simulink library "pd_processing_lib"  (R2018b)
settings: Solver=VariableStepAuto  StartTime=0.0  StopTime=10.0  RelTol=1e-3
settings Model: Creator=Taylor  LastModifiedBy=Taylor

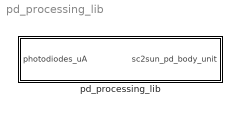
== system pd_processing_lib ==
  pd_processing_lib : Subsystem

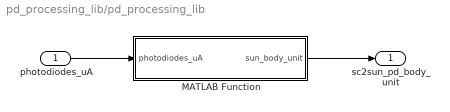
== system pd_processing_lib/pd_processing_lib ==
  photodiodes_uA : Inport
  MATLAB Function : MATLAB Function  TreatAsAtomicUnit=on
  sc2sun_pd_body_unit : Outport
  wires:
  photodiodes_uA/1 -> MATLAB Function/1(photodiodes_uA)
  MATLAB Function/1(sun_body_unit) -> sc2sun_pd_body_unit/1

== matlab function pd_processing_lib/MATLAB Function ==
  data: photodiodes_uA input double size=6; sun_body_unit output double size=3; fswParams parameter
function sun_body_unit = get_sun_body(photodiodes_uA, fswParams)
%GET_SUN_BODY
%
% Estimate the sc2sun vector in the body frame by using photodiode current
% data. 
%
% T. P. Reynolds
%#codegen

normals = [ 1,    -1,     0,     0,     0,     0;
            0,     0,     1,    -1,     0,     0;
            0,     0,     0,     0,     1,    -1 ];
I_thresh_uA = fswParams.controllers.sunseek.I_thresh_uA;

sun_body_unit = zeros(3,1);
for k = 1:6
    if (photodiodes_uA(k) > I_thresh_uA)
        sun_body_unit = sun_body_unit + normals(:,k);
    end
end

if ( norm(sun_body_unit-normals(:,4)) < 1e-8 )
    % sort the amps in ascending order
    [~,ordr_A] = sort(photodiodes_uA);
    % add the second strongest photodiode reading to the estimated sun vector.
    % Because ordr_A is ascending, and there are always 6 entries, the
    % second strongest is always in the 5th location
    sun_body_unit = sun_body_unit + normals(:,ordr_A(5));
end

% if norm(sun_body_unit) < 1 at this point, then none of the if conditions
% above evaluated to true. Therefore, no photodiodes are registering enough
% current, and we assume that the -zB axis [normals(:,6)] has the most
% incidence with the sun vector.
if (norm(sun_body_unit)<1)
    sun_body_unit = normals(:,6);
else
    sun_body_unit = sun_body_unit ./ norm(sun_body_unit);
end

end
